simulink model "Ts"  (R2022b)
settings: Solver=FixedStepAuto  StartTime=0.0  StopTime=10.0  RelTol=1e-3
settings Model: Creator=86134  LastModifiedBy=86134

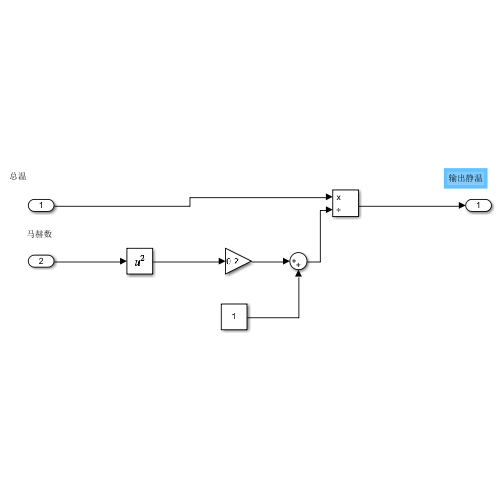
[thumbnail: Simulink's stored preview of the top-level diagram]
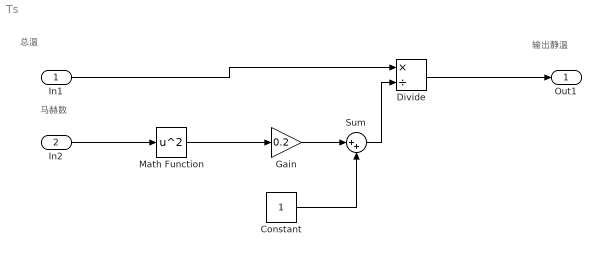
== system Ts ==
  note: 输出静温
  note: 总温
  note: 马赫数
  In1 : Inport
  In2 : Inport  Port=2
  Constant : Constant
  Divide : Product  Inputs=*/
  Gain : Gain  Gain=0.2
  Math Function : Math  Operator=square
  Sum : Sum  Inputs=|++
  Out1 : Outport
  wires:
  In2/1 -> Math Function/1
  Math Function/1 -> Gain/1
  Constant/1 -> Sum/2
  Gain/1 -> Sum/1
  In1/1 -> Divide/1
  Sum/1 -> Divide/2
  Divide/1 -> Out1/1
